simulink model "exec_test"  (Simulink 7.3)
settings: Solver=ode45  StartTime=0.0  StopTime=10.0  RelTol=1e-3
libraries: SimulinkExecutionControl x1
settings Model: Creator=raarenst  LastModifiedBy=raarenst
settings OptimizationCC: InitFltsAndDblsToZero=on
settings DebuggingCC: SaveWithParameterizedLinksMsg=none  SignalResolutionControl=TryResolveAllWithWarning  MultiTaskDSMMsg=warning  MultiTaskCondExecSysMsg=none
settings RTWCC: IncludeERTFirstTime=on
settings GRTTargetCC: TargetFcnLib=ansi_tfl_tmw.mat

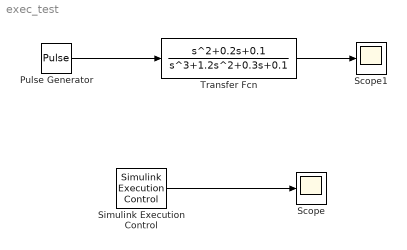
== system exec_test ==
  Pulse Generator : DiscretePulseGenerator  PulseType=Time based  Amplitude=1  Period=1  PulseWidth=50  PhaseDelay=0  SampleTime=1
  Scope : Scope
      settings: YMin=0  YMax=3
  Scope1 : Scope
  Simulink Execution Control : SimulinkExecutionControl/Simulink Execution Control  SystemSampleTime=-1  proc_pri=NORMAL_PRIORITY_CLASS  thread_pri=THREAD_PRIORITY_NORMAL  rt_sim=on  factor=1  ovrrun=Continue execution  Ts=1e-3
  Transfer Fcn : TransferFcn  Numerator=[1 0.2 0.1]  Denominator=[1 1.2 0.3 0.1]
  wires:
  Simulink Execution Control/1 -> Scope/1
  Pulse Generator/1 -> Transfer Fcn/1
  Transfer Fcn/1 -> Scope1/1
